simulink model "pid"  (R2018a)
settings: Solver=VariableStepAuto  StartTime=0.0  StopTime=2000  RelTol=1e-3
settings Model: Creator=Dani  LastModifiedBy=Dani

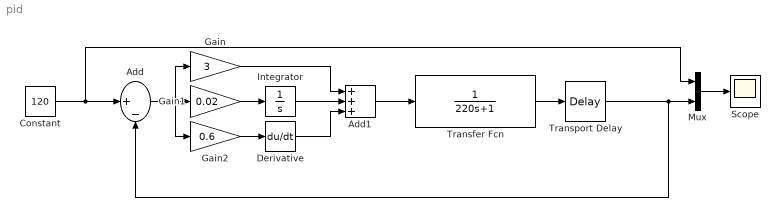
== system pid ==
  Add : Sum  Inputs=|+-
  Add1 : Sum  Inputs=3
  Constant : Constant  Value=120
  Derivative : Derivative  CoefficientInTFapproximation=1
  Gain : Gain  Gain=3
  Gain1 : Gain  Gain=0.02
  Gain2 : Gain  Gain=0.6
  Integrator : Integrator
  Mux : Mux  Inputs=2
  Scope : Scope
  Transfer Fcn : TransferFcn  Denominator=[220 1]
  Transport Delay : TransportDelay  DelayTime=30
  wires:
  Constant/1 -> Add/1, Mux/1
  Transfer Fcn/1 -> Transport Delay/1
  Transport Delay/1 -> Mux/2, Add/2
  Mux/1 -> Scope/1
  Integrator/1 -> Add1/2
  Derivative/1 -> Add1/3
  Add/1 -> Gain2/1, Gain1/1, Gain/1
  Gain/1 -> Add1/1
  Gain1/1 -> Integrator/1
  Gain2/1 -> Derivative/1
  Add1/1 -> Transfer Fcn/1
